simulink library "TrafficSimulationLibrary"  (R2021a)
settings: Solver=VariableStepAuto  StartTime=0.0  StopTime=10.0  RelTol=1e-3
libraries: simulink x1
settings Model: Creator=phill  LastModifiedBy=phill

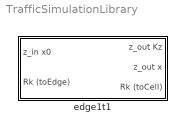
== system TrafficSimulationLibrary ==
  edge1t1 : Subsystem
      settings: PortSchema="{\"entries\":[{\"content\":{\"sides\":[{\"content\":{\"connectorIds\":[\"In1\",\"Out2\"]},\"type\":\"ConnectorPlacement.EquallySpacedRectSide\",\"uuid\":\"c437cf4c-79e4-403f-acc5-73d37113f26d\"},{\"content\":{\"connectorIds\":[\"In2\",\"In3\",\"Out1\"],\"side\":\"RIGHT\"},\"type\":\"ConnectorPlacement.EquallySpacedRectSide\",\"uuid\":\"b2176c48-3cc9-4030-bf6c-6d327e823efa\"},{\"content\":{\"connectorIds\":[],\"side\":\"TOP\"},\"type\":\"ConnectorPlacement.EquallySpacedRectSide\",\"uuid\":\"abeed986-5952-4b96-a6ed-dc33fbc723e6\"}]},\"type\":\"ConnectorPlacement.EquallySpacedConnector\",\"uuid\":\"f01997e7-23a3-4397-8121-8272fdaf74ca\"}],\"packageUris\":[\"http://schema.mathworks.com/mf0/Connector/R2020b\"],\"version\":\"1.0\"}"

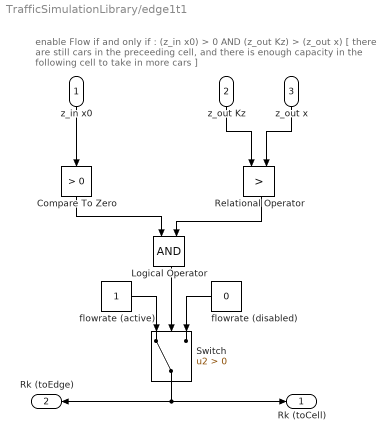
== system TrafficSimulationLibrary/edge1t1 ==
  note: enable Flow if and only if : (z_in x0) > 0 AND (z_out Kz) > (z_out x)
      | [ there are still cars in the preceeding cell, and there is enough capacity
      | in the following cell to take in more cars ]
  z_in x0 : Inport
  z_out Kz : Inport  Port=2
  z_out x : Inport  Port=3
  Compare To Zero : simulink/Logic and Bit Operations/Compare To Zero  relop=>  OutDataTypeStr=boolean
  Logical Operator : Logic  AllPortsSameDT=off  OutDataTypeStr=boolean
  Relational Operator : RelationalOperator  Operator=>  OutDataTypeStr=boolean  RndMeth=Simplest
  Switch : Switch  Criteria=u2 > Threshold
  flowrate (active) : Constant
  flowrate (disabled) : Constant  Value=0
  Rk (toCell) : Outport
  Rk (toEdge) : Outport  Port=2
  wires:
  Switch/1 -> Rk (toCell)/1, Rk (toEdge)/1
  z_out x/1 -> Relational Operator/2
  Relational Operator/1 -> Logical Operator/2
  flowrate (disabled)/1 -> Switch/3
  flowrate (active)/1 -> Switch/1
  z_in x0/1 -> Compare To Zero/1
  Compare To Zero/1 -> Logical Operator/1
  Logical Operator/1 -> Switch/2
  z_out Kz/1 -> Relational Operator/1
